simulink model "assignment_2a"  (R2023b)
settings: Solver=ode4  StartTime=0.0  StopTime=10.0  FixedStep=0.005  RelTol=1e-3
settings Model: Creator=HP  LastModifiedBy=HP

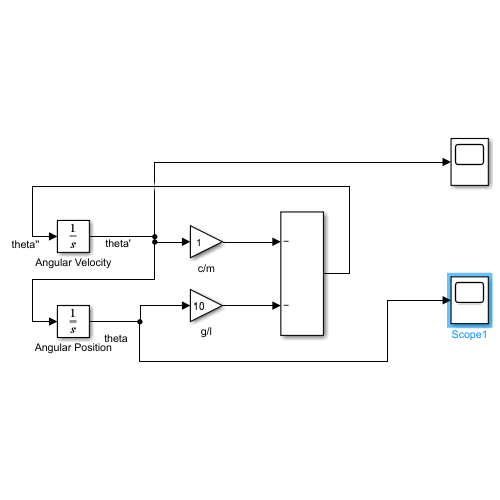
[thumbnail: Simulink's stored preview of the top-level diagram]
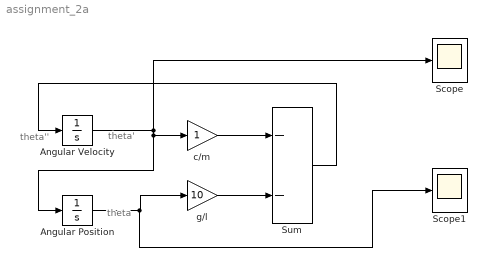
== system assignment_2a ==
  note: theta
  note: theta'
  note: theta''
  Angular Position : Integrator  InitialCondition=0.173648178
  Angular Velocity : Integrator
  Scope : Scope
  Scope1 : Scope
  Sum : Sum  Inputs=--
  c/m : Gain
  g/l : Gain  Gain=10
  wires:
  Sum/1 -> Angular Velocity/1
  Angular Velocity/1 -> Angular Position/1, c/m/1, Scope/1
  c/m/1 -> Sum/1
  g/l/1 -> Sum/2
  Angular Position/1 -> Scope1/1, g/l/1
